simulink model "GuiamentoAtitude"  (R2024a)
settings: Solver=FixedStepAuto  StartTime=0.0  StopTime=tf  FixedStep=step_modelo  RelTol=1e-3
undefined symbols (not defined in the file or in its folder): Re
settings Model: Creator=rodri  LastModifiedBy=rodri
settings DataIOCC: SaveOutput=off  SaveTime=off
settings RTWCC: GPUComputeCapability=3.5

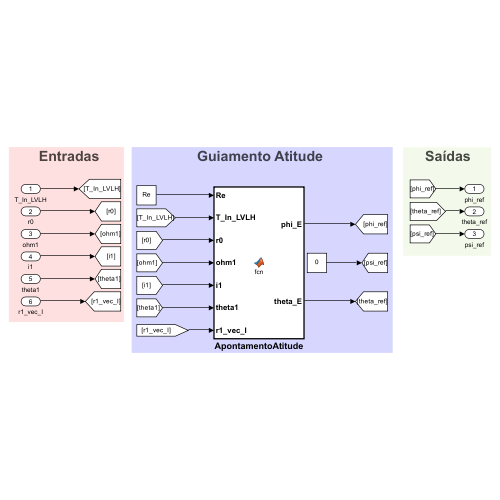
[thumbnail: Simulink's stored preview of the top-level diagram]
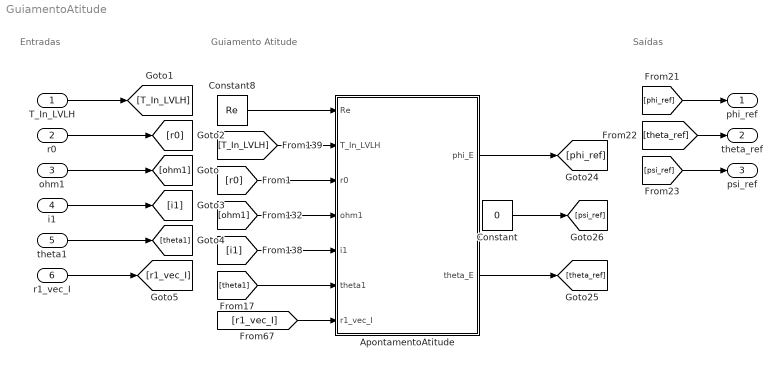
== system GuiamentoAtitude ==
  note: Entradas
  note: Saídas
  note: Guiamento Atitude
  T_In_LVLH : Inport  PortDimensions=[3,3]
  r0 : Inport  Port=2
  ohm1 : Inport  Port=3
  i1 : Inport  Port=4
  theta1 : Inport  Port=5
  r1_vec_I : Inport  Port=6  PortDimensions=[3,1]
  ApontamentoAtitude : MATLAB Function  TreatAsAtomicUnit=on
  Constant : Constant  Value=0  SampleTime=-1
  Constant8 : Constant  Value=Re  SampleTime=-1
  phi_ref : Outport  OutDataTypeStr=double
  theta_ref : Outport  Port=2  OutDataTypeStr=double
  psi_ref : Outport  Port=3  OutDataTypeStr=double
  wires:
  [theta1] -> ApontamentoAtitude/6(theta1)
  Constant8/1 -> ApontamentoAtitude/1(Re)
  [r0] -> ApontamentoAtitude/3(r0)
  [i1] -> ApontamentoAtitude/5(i1)
  [ohm1] -> ApontamentoAtitude/4(ohm1)
  [T_In_LVLH] -> ApontamentoAtitude/2(T_In_LVLH)
  ApontamentoAtitude/2(theta_E) -> [theta_ref]
  [r1_vec_I] -> ApontamentoAtitude/7(r1_vec_I)
  ApontamentoAtitude/1(phi_E) -> [phi_ref]
  T_In_LVLH/1 -> [T_In_LVLH]
  r0/1 -> [r0]
  Constant/1 -> [psi_ref]
  [phi_ref] -> phi_ref/1
  [theta_ref] -> theta_ref/1
  [psi_ref] -> psi_ref/1
  ohm1/1 -> [ohm1]
  i1/1 -> [i1]
  theta1/1 -> [theta1]
  r1_vec_I/1 -> [r1_vec_I]

== matlab function GuiamentoAtitude/ApontamentoAtitude ==
  data: Re input; T_In_LVLH input; r0 input; ohm1 input; i1 input; theta1 input; phi_E output; theta_E output; r1_vec_I input
function [phi_E,theta_E]  = fcn(Re,T_In_LVLH,r0,ohm1,i1,theta1,r1_vec_I)

SO = -r1_vec_I;

r0_vec_I = T_In_LVLH'*[r0 0 0]';

ONl = (r0_vec_I./norm(r0_vec_I)).*Re;
SNl = (SO + ONl);

[T1pi_2,T2pi_2,~] = transfer(pi/2);

[~,T_LVLH_In] = TransInerLVLH(ohm1,theta1,i1);

Fx = T1pi_2*T2pi_2*[1;0;0];
Fx = T_LVLH_In*Fx;

Fx2 = (cross(SO,SNl))/(norm(cross(SO,SNl)));

calc = -(dot(Fx,Fx2)/(norm(Fx)*norm(Fx2)));

if calc >= 1
    calc = 1;
elseif calc <= -1
    calc = -1;
else
    %do nothing
end

phi_E = acos(calc);   %Azimute

%Nesse caso theta é a longitude verdadeira. Para uma órbita não-equatorial,
%estou considerando a longitude verdadeira como a ascensão reta do nodo
%ascendente (ohm) do seguidor.

theta_E = acos(dot(SNl,SO)/(norm(SNl)*norm(SO)));  %Elevation

% LF1 = asin(sin(theta1)*sin(i1));
% 
% if theta1 >=0 && theta1 < pi
%     alphaf1 = acos(cos(theta1/cos(LF1)));
% else
%     alphaf1 = 2*pi - acos(cos(theta1/cos(LF1)));
% end
% 
% 
% alphaf2 = alphaf1 + ohm1;
% LF2 = atan(sin(alphaf2*tan(i0)));
% 
% 
% if theta1 >=0 && theta1 < pi
%     alphaf = acos(cos(LF2*cos(alphaf2)));
% else
%     alphaf = 2*pi - acos(cos(LF2*cos(alphaf2)));
% end
% 
% if alphaf >= 0 && alphaf < pi
%     EL = -acos(dot(FNl,FO)/(norm(FNl)*norm(FO)));
% elseif alphaf >= pi && alphaf <= 2*pi
%     EL = acos(dot(FNl,FO)/(norm(FNl)*norm(FO)));
% else
%     EL = 0;
% end



%% Cálculo das matrizes de transferência
    function [T1,T2,T3] = transfer(alpha)
        T1 = [1 0 0; 0 cos(alpha) sin(alpha); 0 -sin(alpha) cos(alpha)];
        T2 = [cos(alpha) 0 -sin(alpha); 0 1 0; sin(alpha) 0 cos(alpha)];
        T3 = [cos(alpha) sin(alpha) 0; -sin(alpha) cos(alpha) 0; 0 0 1];
    end

end
